simulink model "System_State_Simulation"  (Simulink 6.3)
settings: Solver=VariableStepDiscrete  StartTime=0.0  StopTime=100.0  RelTol=1e-3
libraries: simulink x1
settings Model: LastModifiedBy=Huang

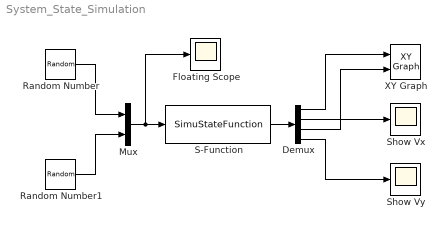
== system System_State_Simulation ==
  Demux : Demux
  Floating Scope : Scope
      settings: TimeRange=10  YMin=-3  YMax=2
  Mux : Mux  Description=Mux  Inputs=2
  Random Number : RandomNumber  Variance=0.01  SampleTime=1
  Random Number1 : RandomNumber  Variance=0.09  Seed=3  SampleTime=1
  S-Function : S-Function  FunctionName=SimuStateFunction
  Show Vx : Scope
  Show Vy : Scope
      settings: SaveName=ScopeData2
  XY Graph : simulink/Sinks/XY Graph  xmin=0  xmax=600  ymin=0  ymax=600  st=1
  wires:
  Random Number/1 -> Mux/1
  Random Number1/1 -> Mux/2
  Mux/1 -> Floating Scope/1, S-Function/1
  S-Function/1 -> Demux/1
  Demux/1 -> XY Graph/1
  Demux/3 -> XY Graph/2
  Demux/4 -> Show Vy/1
  Demux/2 -> Show Vx/1
